simulink model "model_PI_regulator"  (Simulink 7.1)
settings: Solver=ode45  StartTime=0.0  StopTime=20  RelTol=1e-3
settings Model: Creator=ahp  LastModifiedBy=ahp

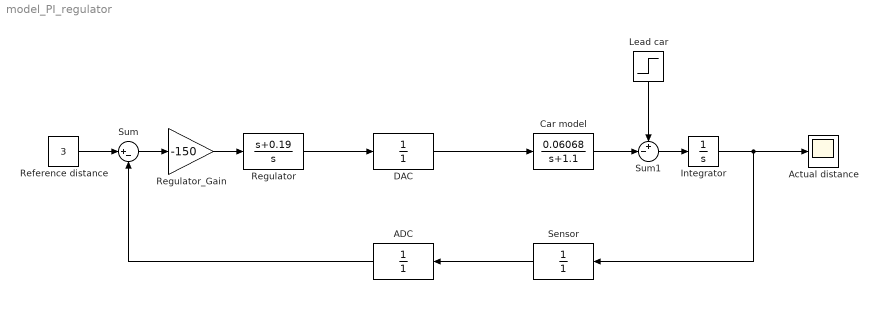
== system model_PI_regulator ==
  ADC : TransferFcn  Orientation=left  Denominator=[1]
  Actual distance : Scope
      settings: YMin=2  YMax=4
  Car model : TransferFcn  Numerator=[0.06068]  Denominator=[1 1.1]
  DAC : TransferFcn  Denominator=[1]
  Integrator : Integrator
  Lead car : Step  Orientation=down  Time=0  SampleTime=0
  Reference distance : Constant  Value=3  OutDataType=sfix(16)  OutScaling=2^0
  Regulator : TransferFcn  Numerator=[1 0.19]  Denominator=[1 0]
  Regulator_Gain : Gain  Gain=-150  ParameterDataType=sfix(16)  ParameterScaling=2^0  OutDataType=sfix(16)  OutScaling=2^0
  Sensor : TransferFcn  Orientation=left  Denominator=[1]
  Sum : Sum  Inputs=|+-  OutDataType=sfix(16)  OutScaling=2^0
  Sum1 : Sum  Inputs=+-|  OutDataType=sfix(16)  OutScaling=2^0
  wires:
  Reference distance/1 -> Sum/1
  Sum/1 -> Regulator_Gain/1
  Car model/1 -> Sum1/2
  Lead car/1 -> Sum1/1
  Sum1/1 -> Integrator/1
  Integrator/1 -> Actual distance/1, Sensor/1
  ADC/1 -> Sum/2
  Regulator/1 -> DAC/1
  DAC/1 -> Car model/1
  Sensor/1 -> ADC/1
  Regulator_Gain/1 -> Regulator/1
